simulink model "boat"  (R2020a)
settings: Solver=VariableStepAuto  StartTime=0.0  StopTime=2*pi  MaxStep=0.02  RelTol=1e-3
undefined symbols (not defined in the file or in its folder): jalla_lqr
settings Model: Creator=g-oft  LastModifiedBy=g-oft

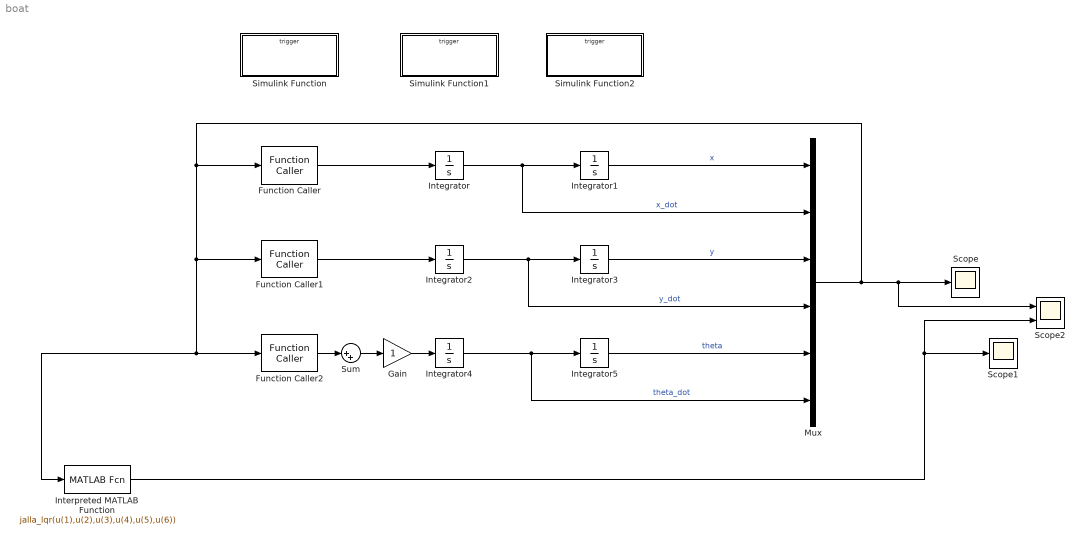
== system boat ==
  Function Caller : FunctionCaller  FunctionPrototype=y = f1(u)  InputArgumentSpecifications=<Enter example>  OutputArgumentSpecifications=<Enter example>
  Function Caller1 : FunctionCaller  FunctionPrototype=y = f2(u)  InputArgumentSpecifications=<Enter example>  OutputArgumentSpecifications=<Enter example>
  Function Caller2 : FunctionCaller  FunctionPrototype=y = f3(u)  InputArgumentSpecifications=<Enter example>  OutputArgumentSpecifications=<Enter example>
  Gain : Gain
  Integrator : Integrator
  Integrator1 : Integrator  InitialCondition=1
  Integrator2 : Integrator  InitialCondition=0.5
  Integrator3 : Integrator
  Integrator4 : Integrator  InitialCondition=0.5
  Integrator5 : Integrator  InitialCondition=pi/2
  Interpreted MATLAB Function : MATLABFcn  MATLABFcn=jalla_lqr(u(1),u(2),u(3),u(4),u(5),u(6))  OutputDimensions=5  Output1D=off
  Mux : Mux  Inputs=6
  Scope : Scope
  Scope1 : Scope
  Scope2 : Scope  NumInputPorts=2
  Simulink Function : Subsystem  TreatAsAtomicUnit=on
  Simulink Function1 : Subsystem  TreatAsAtomicUnit=on
  Simulink Function2 : Subsystem  TreatAsAtomicUnit=on
  Sum : Sum  Inputs=|++
  wires:
  Integrator/1 -> Mux/2, Integrator1/1  "x_dot"
  Integrator2/1 -> Mux/4, Integrator3/1  "y_dot"
  Integrator4/1 -> Mux/6, Integrator5/1  "theta_dot"
  Function Caller/1 -> Integrator/1
  Function Caller1/1 -> Integrator2/1
  Integrator1/1 -> Mux/1  "x"
  Integrator3/1 -> Mux/3  "y"
  Mux/1 -> Function Caller/1, Function Caller1/1, Interpreted MATLAB Function/1, Function Caller2/1, Scope2/1, Scope/1
  Function Caller2/1 -> Sum/1
  Sum/1 -> Gain/1
  Integrator5/1 -> Mux/5  "theta"
  Interpreted MATLAB Function/1 -> Scope2/2, Scope1/1
  Gain/1 -> Integrator4/1

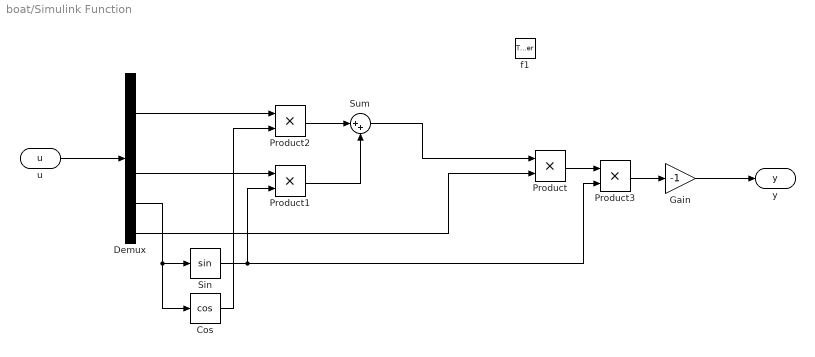
== system boat/Simulink Function ==
  f1 : TriggerPort  TriggerType=function-call  IsSimulinkFunction=on  FunctionName=f1  FunctionVisibility=scoped  VariantControl=(inherit)
  Cos : Trigonometry  Operator=cos
  Demux : Demux  Outputs=6
  Gain : Gain  Gain=-1
  Product{,1..3} (4 alike) : Product
  Sin : Trigonometry
  Sum : Sum  Inputs=|++
  u : ArgIn  DisableCoverage=on  PortDimensions=6  ArgumentName=u
  y : ArgOut  DisableCoverage=on  ArgumentName=y
  wires:
  u/1 -> Demux/1
  Gain/1 -> y/1
  Demux/6 -> Product/2
  Demux/5 -> Cos/1, Sin/1
  Sin/1 -> Product3/2, Product1/2
  Demux/4 -> Product1/1
  Demux/2 -> Product2/1
  Cos/1 -> Product2/2
  Product2/1 -> Sum/1
  Product1/1 -> Sum/2
  Sum/1 -> Product/1
  Product/1 -> Product3/1
  Product3/1 -> Gain/1

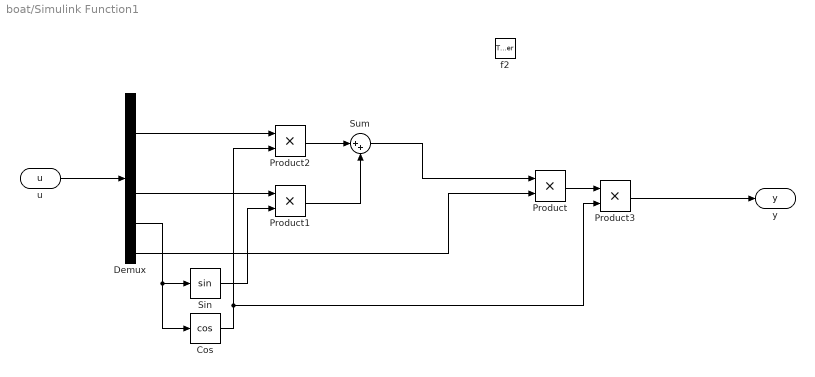
== system boat/Simulink Function1 ==
  f2 : TriggerPort  TriggerType=function-call  IsSimulinkFunction=on  FunctionName=f2  FunctionVisibility=scoped  VariantControl=(inherit)
  Cos : Trigonometry  Operator=cos
  Demux : Demux  Outputs=6
  Product{,1..3} (4 alike) : Product
  Sin : Trigonometry
  Sum : Sum  Inputs=|++
  u : ArgIn  DisableCoverage=on  PortDimensions=6  ArgumentName=u
  y : ArgOut  DisableCoverage=on  ArgumentName=y
  wires:
  Demux/5 -> Cos/1, Sin/1
  Product/1 -> Product3/1
  Product1/1 -> Sum/2
  Cos/1 -> Product3/2, Product2/2
  Sum/1 -> Product/1
  Sin/1 -> Product1/2
  Product2/1 -> Sum/1
  Demux/2 -> Product2/1
  u/1 -> Demux/1
  Product3/1 -> y/1
  Demux/6 -> Product/2
  Demux/4 -> Product1/1

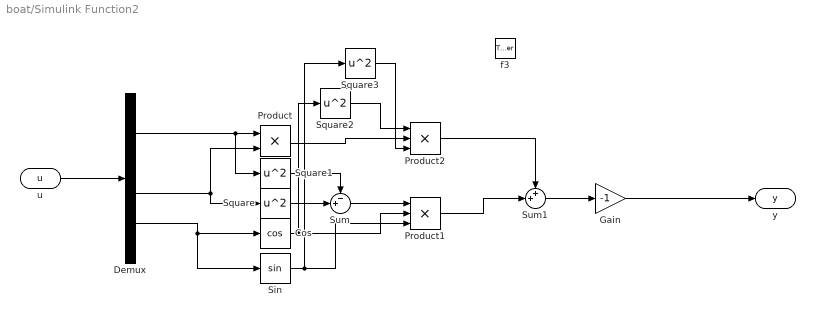
== system boat/Simulink Function2 ==
  f3 : TriggerPort  TriggerType=function-call  IsSimulinkFunction=on  FunctionName=f3  FunctionVisibility=scoped  VariantControl=(inherit)
  Cos : Trigonometry  Operator=cos
  Demux : Demux  Outputs=6
  Gain : Gain  Gain=-1
  Product : Product
  Product1 : Product  Inputs=3
  Product2 : Product  Inputs=***
  Sin : Trigonometry
  Square{,1..3} (4 alike) : Math  Operator=square  SaturateOnIntegerOverflow=on
  Sum : Sum  Inputs=-+|
  Sum1 : Sum  Inputs=++|
  u : ArgIn  DisableCoverage=on  PortDimensions=6  ArgumentName=u
  y : ArgOut  DisableCoverage=on  ArgumentName=y
  wires:
  u/1 -> Demux/1
  Gain/1 -> y/1
  Demux/2 -> Square1/1, Product/1
  Demux/4 -> Square/1, Product/2
  Square/1 -> Sum/2
  Square1/1 -> Sum/1
  Sum/1 -> Product1/1
  Demux/5 -> Sin/1, Cos/1
  Cos/1 -> Square2/1, Product1/2
  Sin/1 -> Square3/1, Product1/3
  Product1/1 -> Sum1/2
  Sum1/1 -> Gain/1
  Product/1 -> Product2/2
  Square2/1 -> Product2/1
  Square3/1 -> Product2/3
  Product2/1 -> Sum1/1
